simulink model "Renewable_Aquarium"  (Simulink 8.3)
settings: Solver=ode3  StartTime=0.0  StopTime=8760  FixedStep=1  MaxStep=1  RelTol=1e-3
values from neighbouring files (symbols this model uses):
  BattC = 500    [Results2 (1).mat]    (also in Results2.mat; RunModel_v2.m)
  batteryEff = 0.98    [Results2 (1).mat]    (also in Results2.mat; RunModel_v2.m)
  cap = 5    [Results2 (1).mat]    (also in Results2.mat; RunModel_v2.m)
  D = [0  5  7  20  22  23.99; 5  10  25  25  10  5]    [Results2 (1).mat]    (also in Results2.mat; RunModel_v2.m = [0 5 7 20 22 23.99; 5 10 25 25 10 5])
  DC = 20    [Results2 (1).mat]    (also in Results2.mat; RunModel_v2.m)
  deltaCap = 0.02    [Results2 (1).mat]    (also in Results2.mat; RunModel_v2.m)
  Dswitch = 0    [Results2 (1).mat]    (also in Results2.mat; RunModel_v2.m)
  ElecC = 0.12    [Results2 (1).mat]    (also in Results2.mat; RunModel_v2.m)
  maxCap = 0.85    [Results2 (1).mat]    (also in Results2.mat; RunModel_v2.m)
  minCap = 0.15    [Results2 (1).mat]    (also in Results2.mat; RunModel_v2.m)
  PanelkWCost = 2500    [Results2 (1).mat]    (also in Results2.mat; RunModel_v2.m)
  PVderating = 0.9    [Results2 (1).mat]    (also in Results2.mat; RunModel_v2.m)
  PVrating = 200    [Results2 (1).mat]    (also in Results2.mat; RunModel_v2.m)
  solarx = 1    [Results2 (1).mat]    (also in Results2.mat; RunModel_v2.m)
  startCap = 0.5    [Results2 (1).mat]    (also in Results2.mat; RunModel_v2.m)
  TurbineCost = 3000    [Results2 (1).mat]    (also in Results2.mat; RunModel_v2.m)
  TurbineCount = 1    [Results2 (1).mat]    (also in Results2.mat; RunModel_v2.m)
  TurbineDerate = 1    [Results2 (1).mat]    (also in Results2.mat; RunModel_v2.m)
  TurbineOpCost = 0    [Results2 (1).mat]    (also in Results2.mat; RunModel_v2.m)
  TurbinePower = [0 3 4 5 6 7 8 9 10 11 12 13 ... (42 elements, 21x2)]    [Results2 (1).mat]    (also in Results2.mat)
  windx = 1    [Results2 (1).mat]    (also in Results2.mat; RunModel_v2.m)
libraries: simulink x6
settings Model: Creator=JACQUELF  LastModifiedBy=Fred
settings DataIOCC: SignalLoggingSaveFormat=Dataset
settings OptimizationCC: ExpressionDepthLimit=2147483647
settings GRTTargetCC: CombineOutputUpdateFcns=on  GRTInterface=off

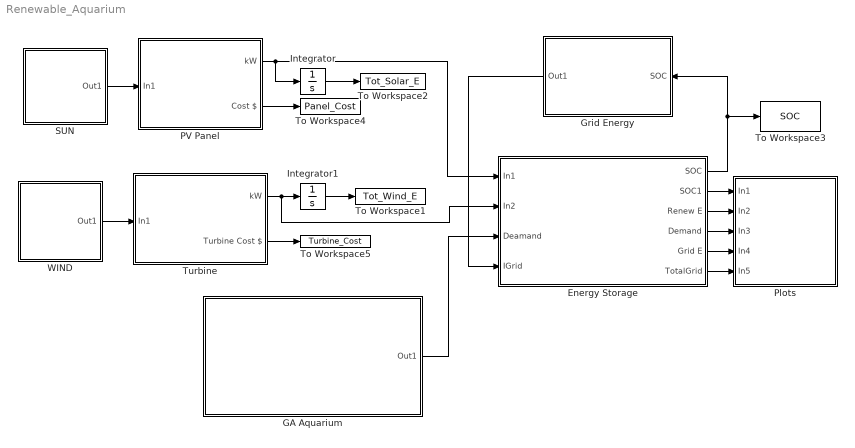
== system Renewable_Aquarium ==
  Energy Storage : Subsystem
      mask Display:
      | image(imread('battery.jpg'))
      | port_label('input', 1, 'PV kW')
      | port_label('input', 2, 'Wind KW')
      | port_label('input', 3, 'Building kW')
      | port_label('input', 4, 'Grid kW')
  GA Aquarium : Subsystem
      mask Display: image(imread('OVTheater3.jpg'))
  Grid Energy : Subsystem
      mask Display: image(imread('grid.jpg'))
  Integrator : Integrator
  Integrator1 : Integrator
  PV Panel : Subsystem
      mask Display:
      | image(imread('PV.jpg'))
      | port_label('output', 1, 'kW')
      | port_label('output', 2, '$')
  Plots : Subsystem
      mask Display: image(imread('plots.jpg'))
  SUN : Subsystem
      mask Display: image(imread('sun.jpg'))
  To Workspace1 : ToWorkspace  VariableName=Tot_Wind_E  SampleTime=-1
  To Workspace2 : ToWorkspace  VariableName=Tot_Solar_E  SampleTime=-1
  To Workspace3 : ToWorkspace  VariableName=SOC  SampleTime=-1
  To Workspace4 : ToWorkspace  VariableName=Panel_Cost  SampleTime=-1
  To Workspace5 : ToWorkspace  VariableName=Turbine_Cost  SampleTime=-1
  Turbine : Subsystem
      mask Display:
      | image(imread('turbine.jpg'))
      | port_label('output', 1, 'kW')
      | port_label('output', 2, '$')
  WIND : Subsystem
      mask Display: image(imread('wind.jpg'))
  wires:
  SUN/1(Out1) -> PV Panel/1(In1)
  PV Panel/1(kW) -> Energy Storage/1(In1), Integrator/1
  WIND/1(Out1) -> Turbine/1(In1)
  Turbine/1(kW) -> Energy Storage/2(In2), Integrator1/1
  Integrator/1 -> To Workspace2/1
  Integrator1/1 -> To Workspace1/1
  Energy Storage/1(SOC) -> To Workspace3/1, Grid Energy/1(SOC)
  PV Panel/2(Cost $) -> To Workspace4/1
  Turbine/2(Turbine Cost $) -> To Workspace5/1
  GA Aquarium/1(Out1) -> Energy Storage/3(Deamand)
  Energy Storage/2(SOC1) -> Plots/1(In1)
  Energy Storage/3(Renew E) -> Plots/2(In2)
  Energy Storage/4(Demand) -> Plots/3(In3)
  Energy Storage/5(Grid E) -> Plots/4(In4)
  Grid Energy/1(Out1) -> Energy Storage/4(IGrid)
  Energy Storage/6(TotalGrid) -> Plots/5(In5)

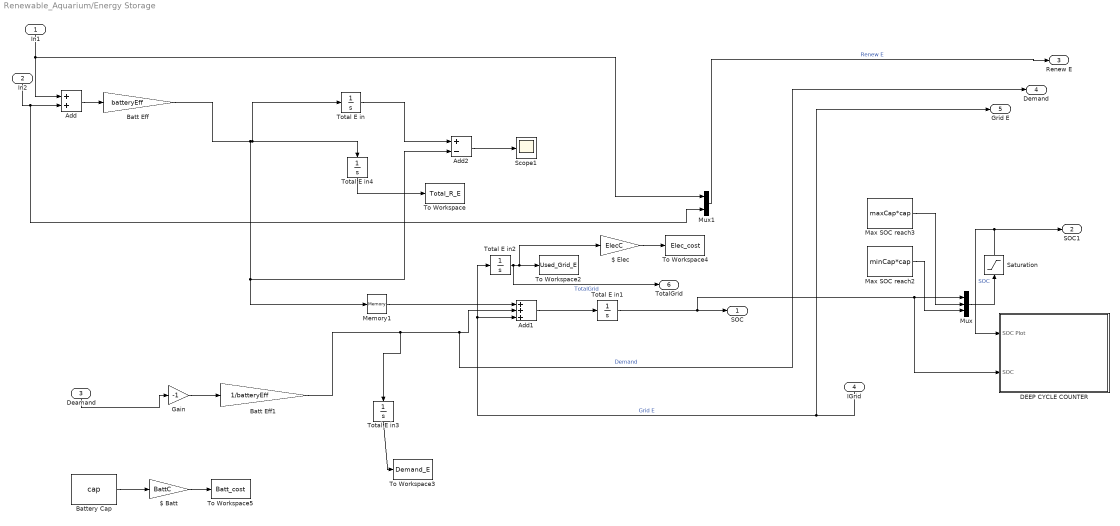
== system Renewable_Aquarium/Energy Storage ==
  In1 : Inport
  In2 : Inport  Port=2
  Deamand : Inport  Port=3
  IGrid : Inport  Port=4
  $ Batt : Gain  Gain=BattC
  $ Elec : Gain  Gain=ElecC
  Add : Sum
  Add1 : Sum  Inputs=+++
  Add2 : Sum  Inputs=+-
  Batt Eff : Gain  Gain=batteryEff
  Batt Eff1 : Gain  Gain=1/batteryEff
  Battery Cap : Constant  Value=cap
  DEEP CYCLE COUNTER : Subsystem
      mask Display: image(imread('counter.jpg'))
  Gain : Gain  Gain=-1
  Max SOC reach2 : Constant  Value=minCap*cap
  Max SOC reach3 : Constant  Value=maxCap*cap
  Memory1 : Memory
  Mux : Mux  Inputs=3
  Mux1 : Mux  Inputs=2
  Saturation : Saturate  UpperLimit=maxCap*cap  LowerLimit=minCap*cap
  Scope1 : Scope
      settings: SaveName=ScopeData2
  To Workspace : ToWorkspace  VariableName=Total_R_E  SampleTime=-1
  To Workspace2 : ToWorkspace  VariableName=Used_Grid_E  SampleTime=-1
  To Workspace3 : ToWorkspace  VariableName=Demand_E  SampleTime=-1
  To Workspace4 : ToWorkspace  VariableName=Elec_cost  SampleTime=-1
  To Workspace5 : ToWorkspace  VariableName=Batt_cost  SampleTime=-1
  Total E in : Integrator
  Total E in1 : Integrator  InitialCondition=startCap*cap  LimitOutput=on  UpperSaturationLimit=maxCap*cap
  Total E in2 : Integrator  UpperSaturationLimit=0.8*cap  LowerSaturationLimit=0
  Total E in3 : Integrator  UpperSaturationLimit=0.8*cap  LowerSaturationLimit=0
  Total E in4 : Integrator  UpperSaturationLimit=0.8*cap  LowerSaturationLimit=0
  SOC : Outport
  SOC1 : Outport  Port=2
  Renew E : Outport  Port=3
  Demand : Outport  Port=4
  Grid E : Outport  Port=5
  TotalGrid : Outport  Port=6
  wires:
  Add/1 -> Batt Eff/1
  Deamand/1 -> Gain/1
  Gain/1 -> Batt Eff1/1
  Total E in/1 -> Add2/1
  Batt Eff/1 -> Total E in4/1, Total E in/1, Add2/2, Memory1/1
  Add2/1 -> Scope1/1
  Memory1/1 -> Add1/1
  Total E in4/1 -> To Workspace/1
  Add1/1 -> Total E in1/1
  $ Elec/1 -> To Workspace4/1
  Battery Cap/1 -> $ Batt/1
  $ Batt/1 -> To Workspace5/1
  Total E in3/1 -> To Workspace3/1
  In1/1 -> Mux1/1, Add/1
  In2/1 -> Mux1/2, Add/2
  Batt Eff1/1 -> Total E in3/1, Demand/1, Add1/2  "Demand"
  IGrid/1 -> Total E in2/1, Add1/3, Grid E/1  "Grid E"
  Max SOC reach3/1 -> Mux/2
  Max SOC reach2/1 -> Mux/3
  Mux/1 -> Saturation/1
  Total E in2/1 -> TotalGrid/1, $ Elec/1, To Workspace2/1  "TotalGrid"
  Mux1/1 -> Renew E/1  "Renew E"
  Saturation/1 -> SOC1/1, DEEP CYCLE COUNTER/1(SOC Plot)  "SOC"
  Total E in1/1 -> DEEP CYCLE COUNTER/2(SOC), Mux/1, SOC/1

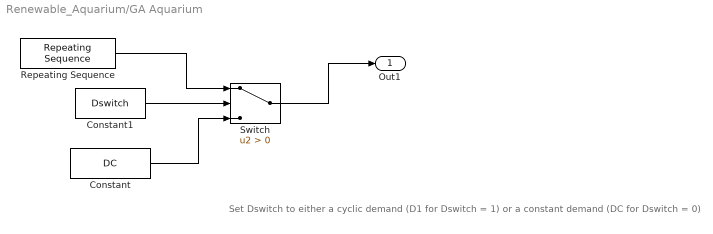
== system Renewable_Aquarium/GA Aquarium ==
  note: Set Dswitch to either a cyclic demand (D1 for Dswitch = 1) or a constant demand (DC for Dswitch = 0)
  Constant : Constant  Value=DC
  Constant1 : Constant  Value=Dswitch
  Repeating Sequence : simulink/Sources/Repeating Sequence  rep_seq_t=D(1,:)  rep_seq_y=D(2,:)
  Switch : Switch  Criteria=u2 > Threshold
  Out1 : Outport
  wires:
  Switch/1 -> Out1/1
  Repeating Sequence/1 -> Switch/1
  Constant/1 -> Switch/3
  Constant1/1 -> Switch/2

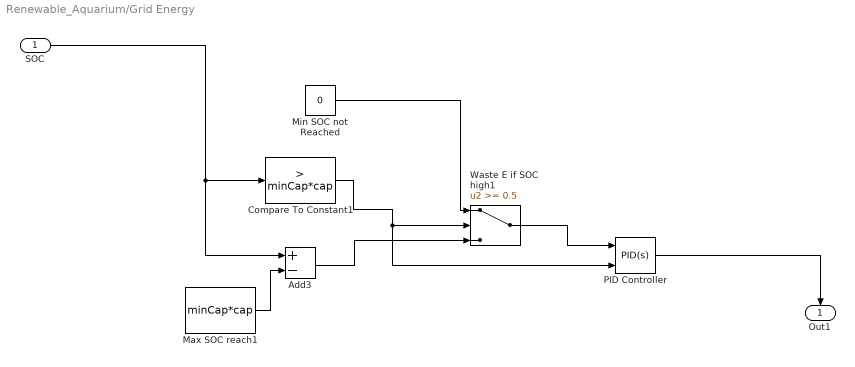
== system Renewable_Aquarium/Grid Energy ==
  SOC : Inport
  Add3 : Sum  Inputs=+-
  Compare To Constant1 : simulink/Logic and Bit Operations/Compare To Constant  relop=>  const=minCap*cap  OutDataTypeStr=boolean
  Max SOC reach1 : Constant  Value=minCap*cap
  Min SOC not Reached : Constant  Value=0
  PID Controller : simulink/Continuous/PID Controller  Controller=PID  TimeDomain=Continuous-time  SampleTime=1  IntegratorMethod=Forward Euler  FilterMethod=Forward Euler  Form=Parallel  P=-1.110  I=-0.15  D=0  N=100  InitialConditionSource=internal  InitialConditionForIntegrator=0  InitialConditionForFilter=0  ExternalReset=rising  LimitOutput=off  UpperSaturationLimit=inf  LowerSaturationLimit=-inf  LinearizeAsGain=on  AntiWindupMode=none  Kb=1  TrackingMode=off  Kt=1  PParamMin=[]  PParamMax=[]  IParamMin=[]  IParamMax=[]  DParamMin=[]  DParamMax=[]  NParamMin=[]  NParamMax=[]  KbParamMin=[]  KbParamMax=[]  KtParamMin=[]  KtParamMax=[]  POutMin=[]  POutMax=[]  IOutMin=[]  IOutMax=[]  DOutMin=[]  DOutMax=[]  NOutMin=[]  NOutMax=[]  KbOutMin=[]  KbOutMax=[]  KtOutMin=[]  KtOutMax=[]  IntegratorOutMin=[]  IntegratorOutMax=[]  FilterOutMin=[]  FilterOutMax=[]  SumOutMin=[]  SumOutMax=[]  SumI1OutMin=[]  SumI1OutMax=[]  SumI2OutMin=[]  SumI2OutMax=[]  SumI3OutMin=[]  SumI3OutMax=[]  SumDOutMin=[]  SumDOutMax=[]  SaturationOutMin=[]  SaturationOutMax=[]  IntegratorContinuousStateAttributes=''  IntegratorStateMustResolveToSignalObject=off  IntegratorRTWStateStorageClass=Auto  FilterContinuousStateAttributes=''  FilterStateMustResolveToSignalObject=off  FilterRTWStateStorageClass=Auto
  Waste E if SOC high1 : Switch  Threshold=0.5
  Out1 : Outport
  wires:
  Min SOC not Reached/1 -> Waste E if SOC high1/1
  Max SOC reach1/1 -> Add3/2
  Compare To Constant1/1 -> PID Controller/2, Waste E if SOC high1/2
  Add3/1 -> Waste E if SOC high1/3
  Waste E if SOC high1/1 -> PID Controller/1
  PID Controller/1 -> Out1/1
  SOC/1 -> Add3/1, Compare To Constant1/1

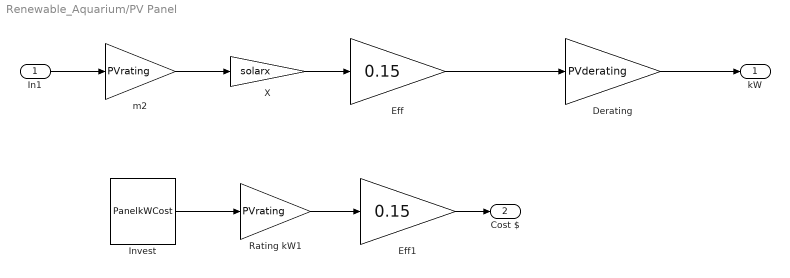
== system Renewable_Aquarium/PV Panel ==
  In1 : Inport
  Derating : Gain  Gain=PVderating
  Eff : Gain  Gain=0.15
  Eff1 : Gain  Gain=0.15
  Invest : Constant  Value=PanelkWCost
  Rating kW1 : Gain  Gain=PVrating
  X : Gain  Gain=solarx
  m2 : Gain  Gain=PVrating
  kW : Outport
  Cost $ : Outport  Port=2
  wires:
  In1/1 -> m2/1
  Derating/1 -> kW/1
  m2/1 -> X/1
  Invest/1 -> Rating kW1/1
  Rating kW1/1 -> Eff1/1
  Eff/1 -> Derating/1
  Eff1/1 -> Cost $/1
  X/1 -> Eff/1

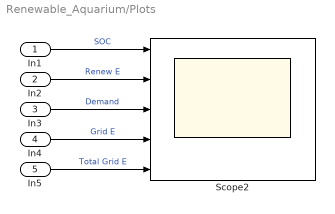
== system Renewable_Aquarium/Plots ==
  In1 : Inport
  In2 : Inport  Port=2
  In3 : Inport  Port=3
  In4 : Inport  Port=4
  In5 : Inport  Port=5
  Scope2 : Scope  NumInputPorts=5
      settings: TimeRange=9000  YMin=0~0~-21.5~0~0  YMax=10~80~-19~25~100000
  wires:
  In1/1 -> Scope2/1  "SOC"
  In2/1 -> Scope2/2  "Renew E"
  In3/1 -> Scope2/3  "Demand"
  In4/1 -> Scope2/4  "Grid E"
  In5/1 -> Scope2/5  "Total Grid E"

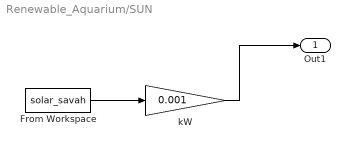
== system Renewable_Aquarium/SUN ==
  From Workspace : FromWorkspace  VariableName=solar_savah  SampleTime=1  Interpolate=off  OutputAfterFinalValue=Holding final value
  kW : Gain  Gain=0.001
  Out1 : Outport
  wires:
  From Workspace/1 -> kW/1
  kW/1 -> Out1/1

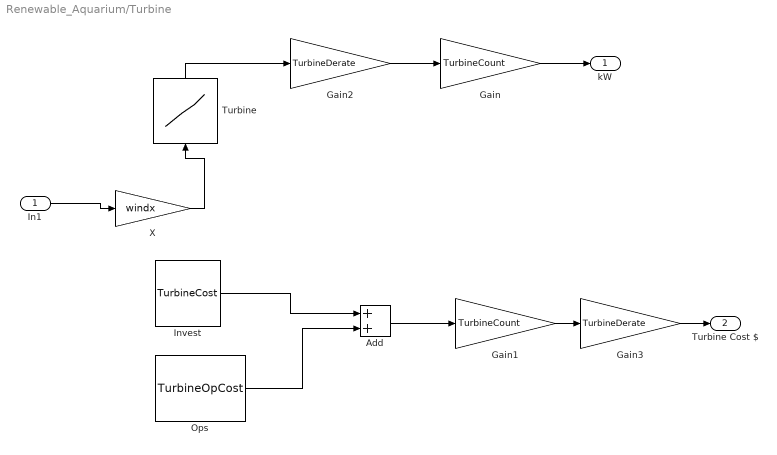
== system Renewable_Aquarium/Turbine ==
  In1 : Inport
  Add : Sum
  Gain : Gain  Gain=TurbineCount
  Gain1 : Gain  Gain=TurbineCount
  Gain2 : Gain  Gain=TurbineDerate
  Gain3 : Gain  Gain=TurbineDerate
  Invest : Constant  Value=TurbineCost
  Ops : Constant  Value=TurbineOpCost
  Turbine : Lookup_n-D  NumberOfTableDimensions=1  BreakpointsForDimension1=TurbinePower(:,1)  Table=TurbinePower(:,2)  ExtrapMethod=Clip  UseLastTableValue=on  RndMeth=Simplest  InputSameDT=on
  X : Gain  Gain=windx
  kW : Outport
  Turbine Cost $ : Outport  Port=2
  wires:
  In1/1 -> X/1
  Turbine/1 -> Gain2/1
  Gain/1 -> kW/1
  Invest/1 -> Add/1
  Ops/1 -> Add/2
  Add/1 -> Gain1/1
  Gain1/1 -> Gain3/1
  Gain2/1 -> Gain/1
  Gain3/1 -> Turbine Cost $/1
  X/1 -> Turbine/1

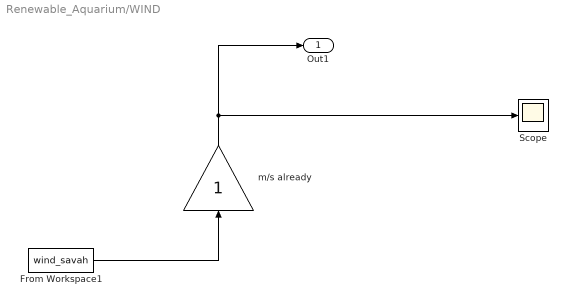
== system Renewable_Aquarium/WIND ==
  " m/s already" : Gain
  From Workspace1 : FromWorkspace  VariableName=wind_savah  SampleTime=1  OutputAfterFinalValue=Holding final value
  Scope : Scope
  Out1 : Outport
  wires:
  From Workspace1/1 -> " m/s already"/1
  " m/s already"/1 -> Scope/1, Out1/1

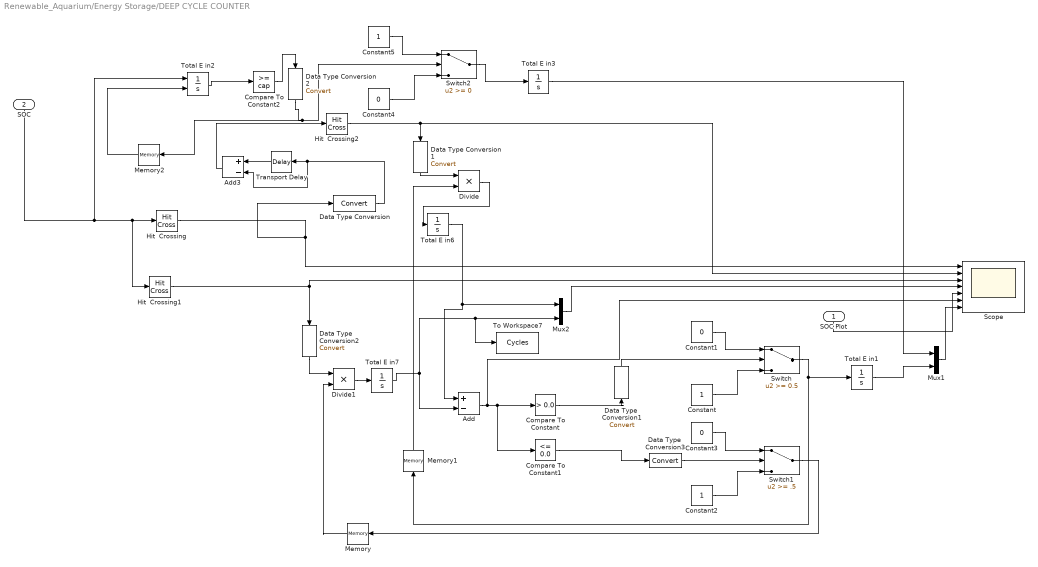
== system Renewable_Aquarium/Energy Storage/DEEP CYCLE COUNTER ==
  SOC Plot : Inport
  SOC : Inport  Port=2
  Add : Sum  Inputs=+-
  Add3 : Sum  Inputs=+-
  Compare To Constant : simulink/Logic and Bit Operations/Compare To Constant  relop=>  const=0.0  OutDataTypeStr=boolean
  Compare To Constant1 : simulink/Logic and Bit Operations/Compare To Constant  relop=<=  const=0.0  OutDataTypeStr=boolean
  Compare To Constant2 : simulink/Logic and Bit Operations/Compare To Constant  relop=>=  const=cap  OutDataTypeStr=boolean
  Constant : Constant
  Constant1 : Constant  Value=0
  Constant2 : Constant
  Constant3 : Constant  Value=0
  Constant4 : Constant  Value=0
  Constant5 : Constant
  Data Type  Conversion1 : DataTypeConversion
  Data Type  Conversion2 : DataTypeConversion
  Data Type  Conversion3 : DataTypeConversion
  Data Type Conversion : DataTypeConversion
  Data Type Conversion1 : DataTypeConversion
  Data Type Conversion2 : DataTypeConversion
  Divide : Product  Inputs=**
  Divide1 : Product  Inputs=**
  Hit  Crossing : HitCross  HitCrossingOffset=(maxCap-deltaCap)*cap  HitCrossingDirection=rising
  Hit  Crossing1 : HitCross  HitCrossingOffset=(minCap+deltaCap)*cap  HitCrossingDirection=falling
  Hit  Crossing2 : HitCross  HitCrossingOffset=1  HitCrossingDirection=rising
  Memory : Memory
  Memory1 : Memory
  Memory2 : Memory
  Mux1 : Mux  Inputs=2
  Mux2 : Mux  Inputs=2
  Scope : Scope  NumInputPorts=7
      settings: TimeRange=9000  YMin=0~0~0~0~0~0~0  YMax=1~1~1~200~6~1~10000  SaveName=ScopeData3
  Switch : Switch  Threshold=0.5
  Switch1 : Switch  Threshold=.5
  Switch2 : Switch
  To Workspace7 : ToWorkspace  VariableName=Cycles  SampleTime=-1
  Total E in{1,3,6..7} (4 alike) : Integrator  UpperSaturationLimit=maxCap*cap
  Total E in2 : Integrator  ExternalReset=rising  UpperSaturationLimit=maxCap*cap
  Transport Delay : TransportDelay
  wires:
  Hit  Crossing/1 -> Data Type Conversion/1, Scope/1
  SOC/1 -> Total E in2/1, Hit  Crossing1/1, Hit  Crossing/1
  SOC Plot/1 -> Scope/5
  Data Type Conversion/1 -> Add3/2, Transport Delay/1
  Transport Delay/1 -> Add3/1
  Mux2/1 -> Scope/4
  Hit  Crossing1/1 -> Scope/3, Data Type  Conversion2/1
  Total E in6/1 -> Add/1, Mux2/1
  Add3/1 -> Hit  Crossing2/1
  Hit  Crossing2/1 -> Data Type Conversion1/1, Scope/2
  Total E in7/1 -> Add/2, To Workspace7/1, Mux2/2
  Add/1 -> Scope/6, Compare To Constant1/1, Compare To Constant/1
  Constant/1 -> Switch/3
  Constant1/1 -> Switch/1
  Constant2/1 -> Switch1/3
  Constant3/1 -> Switch1/1
  Data Type Conversion1/1 -> Divide/1
  Divide/1 -> Total E in6/1
  Compare To Constant/1 -> Data Type  Conversion1/1
  Switch/1 -> Memory1/1, Total E in1/1
  Compare To Constant1/1 -> Data Type  Conversion3/1
  Data Type  Conversion2/1 -> Divide1/1
  Divide1/1 -> Total E in7/1
  Switch1/1 -> Memory/1
  Memory/1 -> Divide1/2
  Memory1/1 -> Divide/2
  Total E in2/1 -> Compare To Constant2/1
  Compare To Constant2/1 -> Data Type Conversion2/1
  Data Type Conversion2/1 -> Switch2/2, Memory2/1
  Constant4/1 -> Switch2/3
  Constant5/1 -> Switch2/1
  Switch2/1 -> Total E in3/1
  Total E in3/1 -> Mux1/1
  Total E in1/1 -> Mux1/2
  Mux1/1 -> Scope/7
  Memory2/1 -> Total E in2/2
  Data Type  Conversion1/1 -> Switch/2
  Data Type  Conversion3/1 -> Switch1/2
